simulink library "PitchController"  (R2023a)
settings: Solver=VariableStepAuto  StartTime=0.0  StopTime=10.0  RelTol=1e-3
undefined symbols (not defined in the file): Pitch
libraries: simulink_extras x5
settings Model: Creator=igmso  LastModifiedBy=igmso

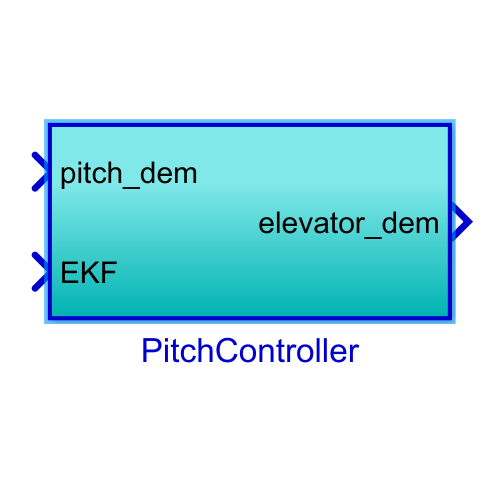
[thumbnail: Simulink's stored preview of the top-level diagram]
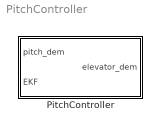
== system PitchController ==
  PitchController : Subsystem  TreatAsAtomicUnit=on  SystemSampleTime=1/Pitch.ControlRate

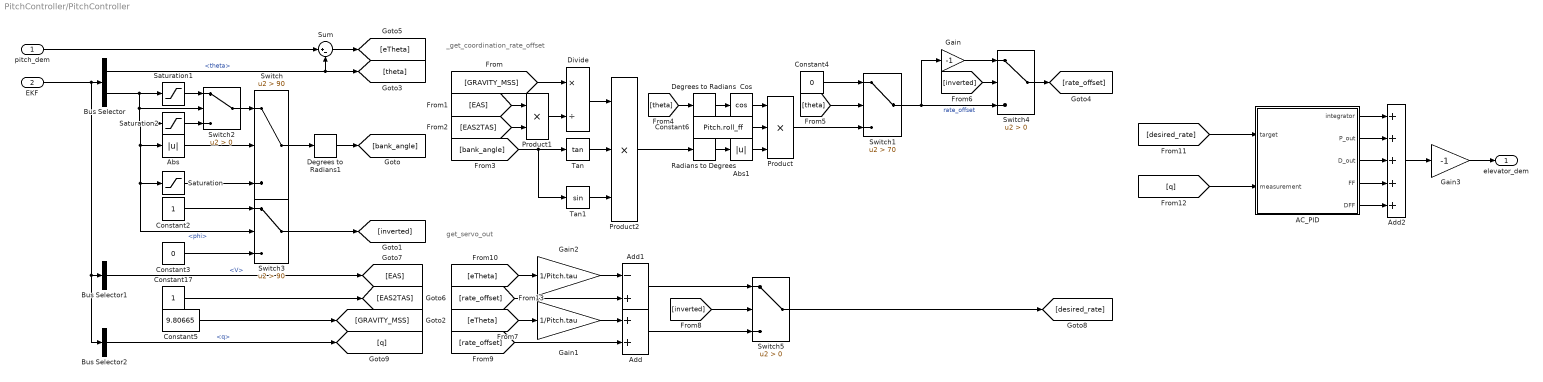
== system PitchController/PitchController ==
  note: _get_coordination_rate_offset
  note: get_servo_out
  pitch_dem : Inport  SampleTime=1/Pitch.ControlRate
  EKF : Inport  Port=2  SampleTime=1/Pitch.ControlRate
  AC_PID : Subsystem
  Abs : Abs  SaturateOnIntegerOverflow=off
  Abs1 : Abs  SaturateOnIntegerOverflow=off
  Add : Sum
  Add1 : Sum  Inputs=-+
  Add2 : Sum  Inputs=5
  Bus Selector : BusSelector  OutputSignals=States.theta,States.phi
  Bus Selector1 : BusSelector  OutputSignals=V
  Bus Selector2 : BusSelector  OutputSignals=States.q
  Constant17 : Constant  SampleTime=1/Pitch.ControlRate
  Constant2 : Constant  SampleTime=1/Pitch.ControlRate
  Constant3 : Constant  Value=0  SampleTime=1/Pitch.ControlRate
  Constant4 : Constant  Value=0  SampleTime=1/Pitch.ControlRate
  Constant5 : Constant  Value=9.80665  SampleTime=1/Pitch.ControlRate
  Constant6 : Constant  Value=Pitch.roll_ff  SampleTime=1/Pitch.ControlRate
  Cos : Trigonometry  Operator=cos
  Degrees to Radians : simulink_extras/Transformations/Degrees to Radians
  Degrees to Radians1 : simulink_extras/Transformations/Degrees to Radians
  Divide : Product  Inputs=*/
  Gain : Gain  Gain=-1
  Gain1 : Gain  Gain=1/Pitch.tau
  Gain2 : Gain  Gain=1/Pitch.tau
  Gain3 : Gain  Gain=-1
  Product : Product  Inputs=3
  Product1 : Product
  Product2 : Product  Inputs=3
  Radians to Degrees : simulink_extras/Transformations/Radians to Degrees
  Saturation : Saturate  UpperLimit=80  LowerLimit=-80
  Saturation1 : Saturate  UpperLimit=180  LowerLimit=100
  Saturation2 : Saturate  UpperLimit=-100  LowerLimit=-180
  Sum : Sum  Inputs=|+-
  Switch : Switch  Criteria=u2 > Threshold  Threshold=90  SaturateOnIntegerOverflow=off  InputSameDT=off
  Switch1 : Switch  Criteria=u2 > Threshold  Threshold=70  SaturateOnIntegerOverflow=off  InputSameDT=off
  Switch2 : Switch  Criteria=u2 > Threshold  SaturateOnIntegerOverflow=off  InputSameDT=off
  Switch3 : Switch  Criteria=u2 > Threshold  Threshold=90  SaturateOnIntegerOverflow=off  InputSameDT=off
  Switch4 : Switch  Criteria=u2 > Threshold  SaturateOnIntegerOverflow=off  InputSameDT=off
  Switch5 : Switch  Criteria=u2 > Threshold  SaturateOnIntegerOverflow=off  InputSameDT=off
  Tan : Trigonometry  Operator=tan
  Tan1 : Trigonometry
  elevator_dem : Outport  SampleTime=1/Pitch.ControlRate
  wires:
  AC_PID/2(P_out) -> Add2/2
  AC_PID/5(DFF) -> Add2/5
  AC_PID/3(D_out) -> Add2/3
  Gain3/1 -> elevator_dem/1
  Add2/1 -> Gain3/1
  AC_PID/4(FF) -> Add2/4
  Bus Selector1/1 -> [EAS]  "<V>"
  Add1/1 -> Switch5/1
  Saturation/1 -> Switch/3
  [eTheta] -> Gain1/1
  [eTheta] -> Gain2/1
  Cos/1 -> Product/1
  Abs/1 -> Switch/2
  [desired_rate] -> AC_PID/1(target)
  Gain2/1 -> Add1/1
  Bus Selector/2 -> Saturation1/1, Switch2/2, Saturation2/1, Abs/1, Saturation/1, Switch3/2  "<phi>"
  Constant6/1 -> Product/2
  Constant4/1 -> Switch1/1
  Constant2/1 -> Switch3/1
  Tan1/1 -> Product2/3
  Gain/1 -> Switch4/1
  [rate_offset] -> Add1/2
  Product/1 -> Switch1/3
  [theta] -> Switch1/2
  Divide/1 -> Product2/1
  [GRAVITY_MSS] -> Divide/1
  [bank_angle] -> Tan/1, Tan1/1
  Bus Selector2/1 -> [q]  "<q>"
  [rate_offset] -> Add/2
  Switch4/1 -> [rate_offset]
  pitch_dem/1 -> Sum/1
  Gain1/1 -> Add/1
  Saturation1/1 -> Switch2/1
  Switch/1 -> Degrees to Radians1/1
  Product1/1 -> Divide/2
  [EAS2TAS] -> Product1/2
  [inverted] -> Switch5/2
  Switch1/1 -> Switch4/3, Gain/1  "rate_offset"
  [theta] -> Degrees to Radians/1
  [q] -> AC_PID/2(measurement)
  Switch3/1 -> [inverted]
  Bus Selector/1 -> [theta], Sum/2  "<theta>"
  [EAS] -> Product1/1
  Switch5/1 -> [desired_rate]
  Switch2/1 -> Switch/1
  Constant17/1 -> [EAS2TAS]
  Degrees to Radians/1 -> Cos/1
  Saturation2/1 -> Switch2/3
  Tan/1 -> Product2/2
  Constant5/1 -> [GRAVITY_MSS]
  Product2/1 -> Radians to Degrees/1
  Sum/1 -> [eTheta]
  [inverted] -> Switch4/2
  EKF/1 -> Bus Selector/1, Bus Selector1/1, Bus Selector2/1
  Degrees to Radians1/1 -> [bank_angle]
  Constant3/1 -> Switch3/3
  Radians to Degrees/1 -> Abs1/1
  AC_PID/1(integrator) -> Add2/1
  Abs1/1 -> Product/3
  Add/1 -> Switch5/3

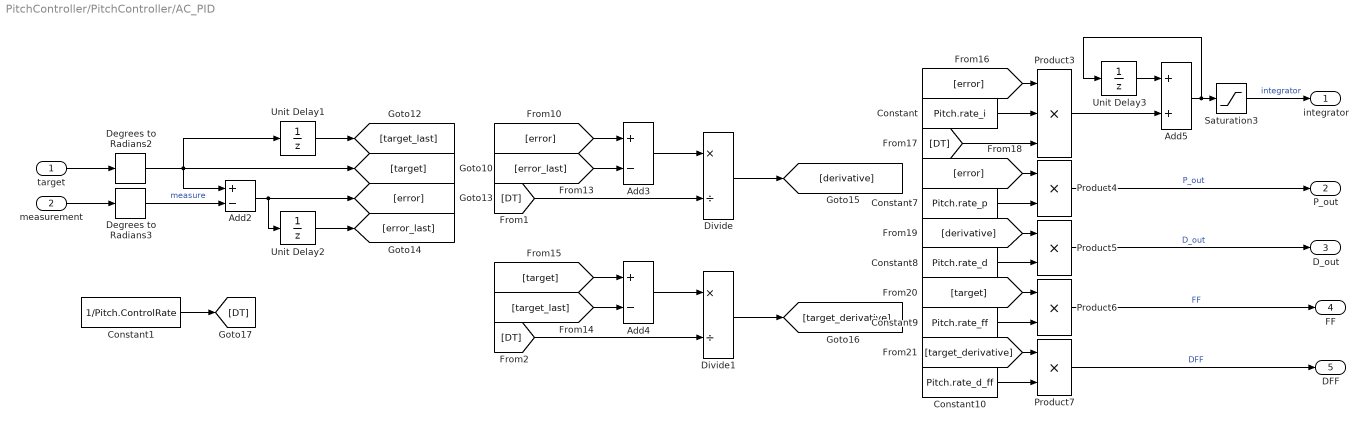
== system PitchController/PitchController/AC_PID ==
  target : Inport
  measurement : Inport  Port=2
  Add2 : Sum  Inputs=+-
  Add3 : Sum  Inputs=+-
  Add4 : Sum  Inputs=+-
  Add5 : Sum
  Constant : Constant  Value=Pitch.rate_i  SampleTime=1/Pitch.ControlRate
  Constant1 : Constant  Value=1/Pitch.ControlRate  SampleTime=1/Pitch.ControlRate
  Constant10 : Constant  Value=Pitch.rate_d_ff  SampleTime=1/Pitch.ControlRate
  Constant7 : Constant  Value=Pitch.rate_p  SampleTime=1/Pitch.ControlRate
  Constant8 : Constant  Value=Pitch.rate_d  SampleTime=1/Pitch.ControlRate
  Constant9 : Constant  Value=Pitch.rate_ff  SampleTime=1/Pitch.ControlRate
  Degrees to Radians2 : simulink_extras/Transformations/Degrees to Radians
  Degrees to Radians3 : simulink_extras/Transformations/Degrees to Radians
  Divide : Product  Inputs=*/
  Divide1 : Product  Inputs=*/
  Product3 : Product  Inputs=3
  Product{4..7} (4 alike) : Product
  Saturation3 : Saturate  UpperLimit=Pitch.rate_imax  LowerLimit=-Pitch.rate_imax
  Unit Delay1 : UnitDelay  SampleTime=1/Pitch.ControlRate  StateName=target_last  HasFrameUpgradeWarning=on
  Unit Delay2 : UnitDelay  SampleTime=1/Pitch.ControlRate  StateName=error_last  HasFrameUpgradeWarning=on
  Unit Delay3 : UnitDelay  SampleTime=1/Pitch.ControlRate  StateName=integrator  HasFrameUpgradeWarning=on
  integrator : Outport
  P_out : Outport  Port=2
  D_out : Outport  Port=3
  FF : Outport  Port=4
  DFF : Outport  Port=5
  wires:
  Constant10/1 -> Product7/2
  Add3/1 -> Divide/1
  [derivative] -> Product5/1
  [target_derivative] -> Product7/1
  [DT] -> Product3/3
  Add2/1 -> Unit Delay2/1, [error]
  Unit Delay3/1 -> Add5/1
  Product7/1 -> DFF/1  "DFF"
  Unit Delay1/1 -> [target_last]
  Degrees to Radians2/1 -> [target], Unit Delay1/1, Add2/1
  Constant9/1 -> Product6/2
  Product4/1 -> P_out/1  "P_out"
  [target] -> Add4/1
  Constant7/1 -> Product4/2
  measurement/1 -> Degrees to Radians3/1
  Saturation3/1 -> integrator/1  "integrator"
  Constant1/1 -> [DT]
  Product3/1 -> Add5/2
  Add5/1 -> Unit Delay3/1, Saturation3/1
  Degrees to Radians3/1 -> Add2/2  "measure"
  [target_last] -> Add4/2
  [error_last] -> Add3/2
  Product5/1 -> D_out/1  "D_out"
  Add4/1 -> Divide1/1
  Product6/1 -> FF/1  "FF"
  Constant8/1 -> Product5/2
  Unit Delay2/1 -> [error_last]
  [target] -> Product6/1
  target/1 -> Degrees to Radians2/1
  Constant/1 -> Product3/2
  [error] -> Product4/1
  [error] -> Product3/1
  [error] -> Add3/1
  Divide/1 -> [derivative]
  [DT] -> Divide/2
  [DT] -> Divide1/2
  Divide1/1 -> [target_derivative]
